simulink model "DC_Motor_control_Direction_3Push_Button"  (R2024a)
settings: Solver=FixedStepDiscrete  StartTime=0.0  StopTime=inf  FixedStep=1e-3  RelTol=1e-3  EnableMultiTasking=on
libraries: arduinolib x6
settings Model: ExtModeTrigDuration=2  Creator=DELL  LastModifiedBy=DELL
settings SolverCC: AutoInsertRateTranBlk=on
settings OptimizationCC: EnhancedBackFolding=on  PassReuseOutputArgsAs=Individual arguments  ZeroExternalMemoryAtStartup=off  ZeroInternalMemoryAtStartup=off  MaxStackSize=64  OptimizeBlockOrder=speed  DifferentSizesBufferReuse=on  OptimizationCustomize=off  EfficientTunableParamExpr=on
settings DebuggingCC: ParameterTunabilityLossMsg=error
settings HardwareCC: ProdBitPerInt=16  ProdBitPerPointer=16  ProdBitPerSizeT=16  ProdBitPerPtrDiffT=16  ProdLargestAtomicFloat=None  ProdWordSize=8  ProdHWDeviceType=Atmel->AVR
settings SFSimCC: MATLABDynamicMemAlloc=off
settings RTWCC: Description=Embedded Coder  SystemTargetFile=ert.tlc  HardwareBoard=Arduino Uno  TemplateMakefile=ert_default_tmf  Toolchain=Arduino AVR  BuildConfiguration=Faster Runs
settings CodeAppCC: ForceParamTrailComments=on  IgnoreCustomStorageClasses=off  OperatorAnnotations=on  SimulinkDataObjDesc=on  SFDataObjDesc=on  InsertBlockDesc=on
settings ERTTargetCC: SupportContinuousTime=on  SupportVariableSizeSignals=on  ExtModeTransport=3  ExtModeStaticAlloc=on  ExtModeAutomaticAllocSize=off  ExtModeStaticAllocSize=250  ExtModeMexFile=ext_xcp  ExtModeIntrfLevel=Level2 - Open

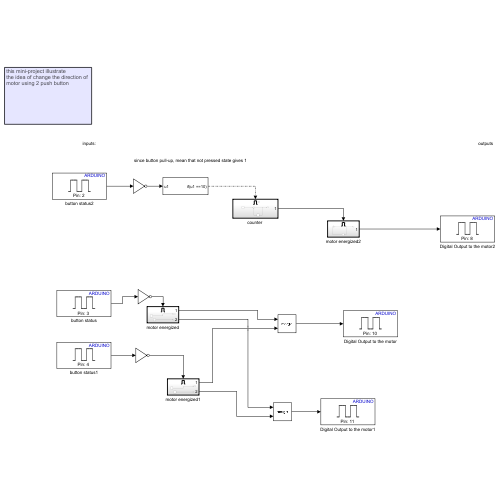
[thumbnail: Simulink's stored preview of the top-level diagram]
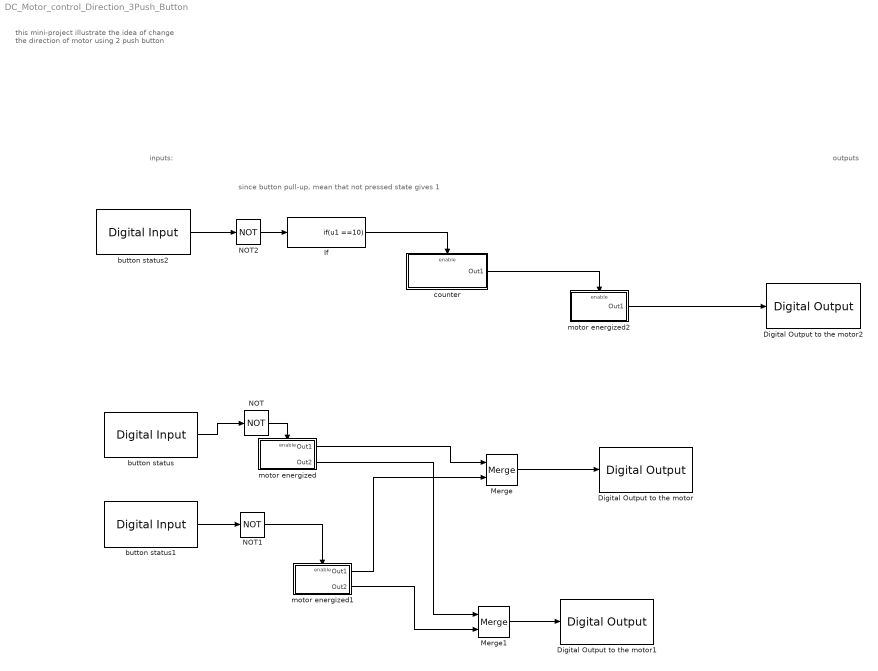
== system DC_Motor_control_Direction_3Push_Button ==
  note: outputs
  note: inputs:
  note: this mini-project illustrate
      | the idea of change the direction of
      | motor using 2 push button
  note: since button pull-up, mean that not pressed state gives 1
  Digital Output to the motor : arduinolib/Digital Output  pinNumber=10  Direction=output  blockPlatform=arduino
  Digital Output to the motor1 : arduinolib/Digital Output  pinNumber=11  Direction=output  blockPlatform=arduino
  Digital Output to the motor2 : arduinolib/Digital Output  pinNumber=8  Direction=output  blockPlatform=arduino
  If : If  IfExpression=u1 ==10  ShowElse=off
  Merge : Merge
  Merge1 : Merge
  NOT : Logic  Operator=NOT  IconShape=distinctive  AllPortsSameDT=off  OutDataTypeStr=boolean
  NOT1 : Logic  Operator=NOT  IconShape=distinctive  AllPortsSameDT=off  OutDataTypeStr=boolean
  NOT2 : Logic  Operator=NOT  IconShape=distinctive  AllPortsSameDT=off  OutDataTypeStr=boolean
  button status : arduinolib/Digital Input  pinNumber=3  mode=Input Pullup  Direction=input  SampleTime=0.1  blockPlatform=arduino
  button status1 : arduinolib/Digital Input  pinNumber=4  mode=Input Pullup  Direction=input  SampleTime=0.1  blockPlatform=arduino
  button status2 : arduinolib/Digital Input  pinNumber=2  mode=Input Pullup  Direction=input  SampleTime=0.1  blockPlatform=arduino
  "counter " : Subsystem  TreatAsAtomicUnit=on
  motor energized : Subsystem  TreatAsAtomicUnit=on
  motor energized1 : Subsystem  TreatAsAtomicUnit=on
  motor energized2 : Subsystem  TreatAsAtomicUnit=on
  wires:
  button status/1 -> NOT/1
  button status1/1 -> NOT1/1
  Merge/1 -> Digital Output to the motor/1
  Merge1/1 -> Digital Output to the motor1/1
  NOT/1 -> motor energized/Enable
  NOT1/1 -> motor energized1/Enable
  motor energized/1(Out1) -> Merge/1
  motor energized/2(Out2) -> Merge1/1
  motor energized1/1(Out1) -> Merge/2
  motor energized1/2(Out2) -> Merge1/2
  motor energized2/1(Out1) -> Digital Output to the motor2/1
  button status2/1 -> NOT2/1
  If/1 -> "counter "/Enable
  NOT2/1 -> If/1
  "counter "/1(Out1) -> motor energized2/Enable

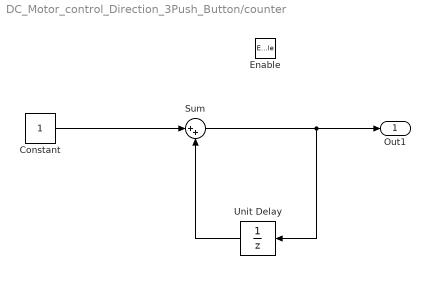
== system DC_Motor_control_Direction_3Push_Button/counter  ==
  Enable : EnablePort  StatesWhenEnabling=reset
  Constant : Constant
  Sum : Sum  Inputs=|++
  Unit Delay : UnitDelay  SampleTime=-1  HasFrameUpgradeWarning=on
  Out1 : Outport
  wires:
  Unit Delay/1 -> Sum/2
  Constant/1 -> Sum/1
  Sum/1 -> Unit Delay/1, Out1/1

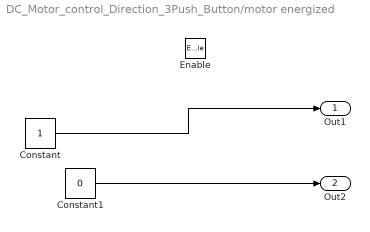
== system DC_Motor_control_Direction_3Push_Button/motor energized ==
  Enable : EnablePort
  Constant : Constant
  Constant1 : Constant  Value=0
  Out1 : Outport
  Out2 : Outport  Port=2
  wires:
  Constant/1 -> Out1/1
  Constant1/1 -> Out2/1

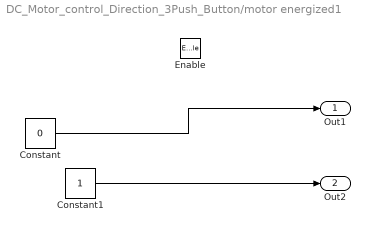
== system DC_Motor_control_Direction_3Push_Button/motor energized1 ==
  Enable : EnablePort
  Constant : Constant  Value=0
  Constant1 : Constant
  Out1 : Outport
  Out2 : Outport  Port=2
  wires:
  Constant1/1 -> Out2/1
  Constant/1 -> Out1/1

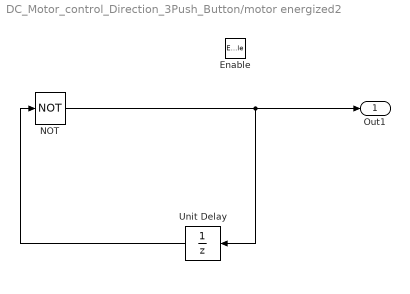
== system DC_Motor_control_Direction_3Push_Button/motor energized2 ==
  Enable : EnablePort
  NOT : Logic  Operator=NOT  IconShape=distinctive  AllPortsSameDT=off  OutDataTypeStr=boolean
  Unit Delay : UnitDelay  SampleTime=-1  HasFrameUpgradeWarning=on
  Out1 : Outport
  wires:
  Unit Delay/1 -> NOT/1
  NOT/1 -> Unit Delay/1, Out1/1
